simulink model "Simulink_8"  (R2024b)
settings: Solver=ode15s  StartTime=0.0  StopTime=15  RelTol=1e-3
undefined symbols (not defined in the file): C2, C4, C6, qhome
libraries: robotmaniplib x2, simulink x1, robotcorelib x1
settings Model: Creator=jaekel  LastModifiedBy=ACKDE
settings DataIOCC: InspectSignalLogs=on
settings RTWCC: GPUComputeCapability=3.5

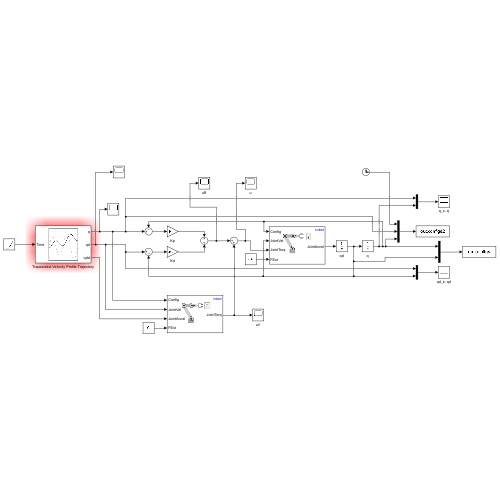
[thumbnail: Simulink's stored preview of the top-level diagram]
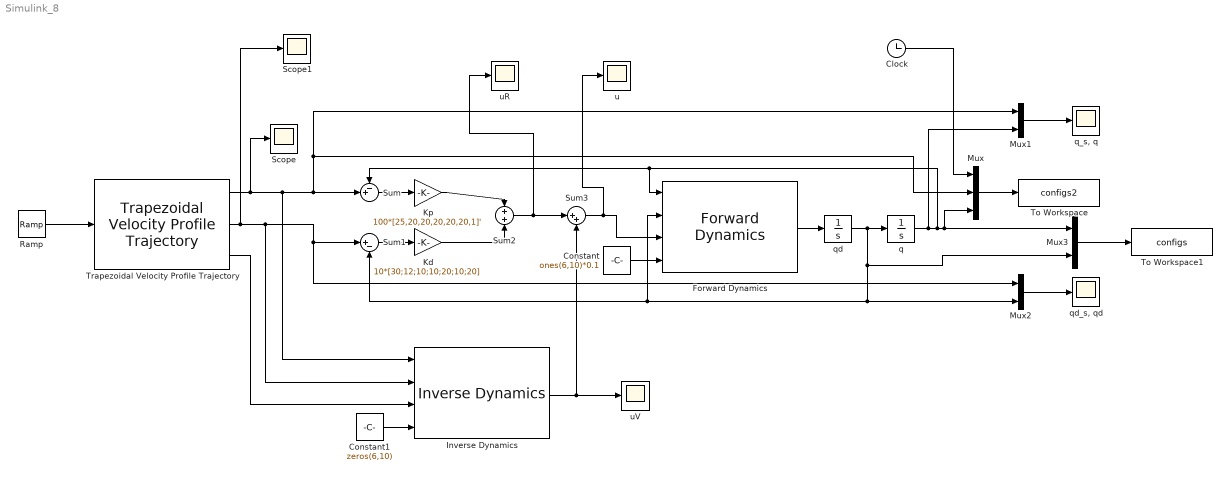
== system Simulink_8 ==
  Clock : Clock
  Constant : Constant  Value=ones(6,10)*0.1
  Constant1 : Constant  Value=zeros(6,10)
  Forward Dynamics : robotmaniplib/Forward Dynamics  RigidBodyTree=robot  SimulateUsing=Interpreted execution
  Inverse Dynamics : robotmaniplib/Inverse Dynamics  RigidBodyTree=robot  SimulateUsing=Interpreted execution
  Kd : Gain  Gain=10*[30;12;10;10;20;10;20]
  Kp : Gain  Gain=100*[25,20,20,20,20,20,1]'
  Mux : Mux  Inputs=3
  Mux1 : Mux  Inputs=2
  Mux2 : Mux  Inputs=2
  Mux3 : Mux  Inputs=2
  Ramp : simulink/Sources/Ramp  slope=1  start=0  InitialOutput=0
  Scope : Scope
  Scope1 : Scope
  Sum : Sum  Inputs=-+|
  Sum1 : Sum  Inputs=|+-
  Sum2 : Sum  Inputs=+|+
  Sum3 : Sum  Inputs=|++
  To Workspace : ToWorkspace  VariableName=configs2  SampleTime=-1
  To Workspace1 : ToWorkspace  VariableName=configs  SampleTime=-1
  Trapezoidal Velocity Profile Trajectory : robotcorelib/Trapezoidal Velocity Profile Trajectory  WaypointSource=Internal  Waypoints=[qhome',C1',C2',C3',C4',C5',C6',C7']  NumParams=1  Parameter1=End Time  Parameter2=End Time  ParameterSource=Internal  PeakVelocity=[ 2; 2 ]  Acceleration=[ 1; 2 ]  EndTime=2  AccelTime=[ 1; 2 ]  SimulateUsing=Interpreted execution
  q : Integrator  InitialCondition=qhome
  "q_s, q" : Scope
  qd : Integrator
  "qd_s, qd" : Scope
  u : Scope
  uR : Scope
  uV : Scope
  wires:
  Trapezoidal Velocity Profile Trajectory/1 -> Scope/1, Inverse Dynamics/1, Sum/2, Mux/2, Mux1/1
  Trapezoidal Velocity Profile Trajectory/2 -> Scope1/1, Sum1/1, Mux2/1, Inverse Dynamics/2
  Ramp/1 -> Trapezoidal Velocity Profile Trajectory/1
  Mux1/1 -> "q_s, q"/1
  Mux/1 -> To Workspace/1
  Clock/1 -> Mux/1
  Mux2/1 -> "qd_s, qd"/1
  Forward Dynamics/1 -> qd/1
  qd/1 -> Mux3/2, Mux2/2, Sum1/2, Forward Dynamics/2, q/1
  q/1 -> Mux1/2, Forward Dynamics/1, Sum/1, Mux3/1, Mux/3
  Constant/1 -> Forward Dynamics/4
  Sum/1 -> Kp/1
  Sum1/1 -> Kd/1
  Kp/1 -> Sum2/1
  Kd/1 -> Sum2/2
  Sum3/1 -> u/1, Forward Dynamics/3
  Inverse Dynamics/1 -> Sum3/2, uV/1
  Constant1/1 -> Inverse Dynamics/4
  Trapezoidal Velocity Profile Trajectory/3 -> Inverse Dynamics/3
  Sum2/1 -> uR/1, Sum3/1
  Mux3/1 -> To Workspace1/1
